simulink model "Delay_Without_Delay"  (R2025b)
settings: Solver=FixedStepDiscrete  StartTime=0.0  StopTime=10.0  FixedStep=0.01  RelTol=1e-3
libraries: simulink x1
settings Model: Creator=soura  LastModifiedBy=soura

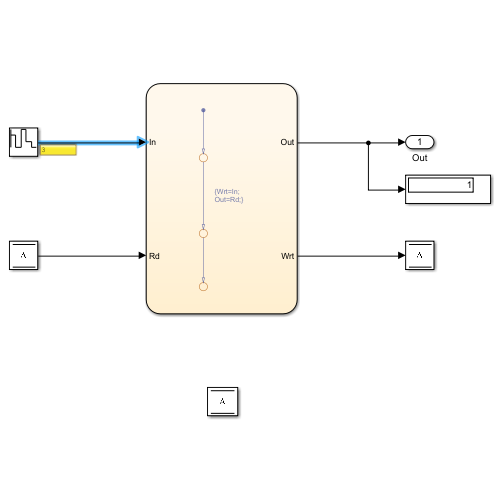
[thumbnail: Simulink's stored preview of the top-level diagram]
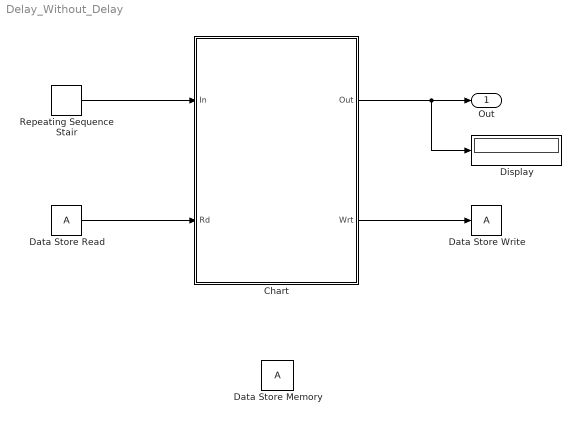
== system Delay_Without_Delay ==
  Chart : Stateflow chart  TreatAsAtomicUnit=on
  Data Store Memory : DataStoreMemory  WriteAfterWriteMsg=warning  InitialValue=7  ShowAdditionalParam=off
  Data Store Read : DataStoreRead  IndexOptions=Index vector (dialog)  Indices=1  OutputSizes=1
  Data Store Write : DataStoreWrite  IndexOptions=Index vector (dialog)  Indices=1  OutputSizes=1
  Display : Display
  Repeating Sequence Stair : simulink/Sources/Repeating Sequence Stair  OutValues=[3 1 4 2 1].'  tsamp=-1  OutMin=[]  OutMax=[]  OutDataTypeStr=double  OutputDataTypeScalingMode=double  OutDataType=fixdt(0,8)  ConRadixGroup=Best Precision: Vector-wise  OutScaling=2^-12
  Out : Outport
  wires:
  Repeating Sequence Stair/1 -> Chart/1(In)
  Data Store Read/1 -> Chart/2(Rd)
  Chart/1(Out) -> Display/1, Out/1
  Chart/2(Wrt) -> Data Store Write/1

== stateflow chart Delay_Without_Delay/Chart ==
  (default) -> (junction 1)
  (junction 1) -> (junction 5) : {Wrt=In;
      | Out=Rd;}
  (junction 5) -> (junction 6)
  data: In input; Rd input; Out output; Wrt output
